simulink model "HVDCMTGW"  (R2025b)
settings: Solver=VariableStepAuto  StartTime=0.0  StopTime=Tsim  FixedStep=5e-5  RelTol=1e-3
PreLoadFcn:
  | SimulationTime = 3.5;
  | HVDCParameters;
  | Tsim = 3.5;
undefined symbols (not defined in the file): base, Base, Connection1, Connection2, Connection3, DiscIntNeverNeededParam, ee_sli_rtmsupport, frt, gcbh, grid, HVDC, lvrt, onshoreGfm, pll, pmsm, PVController, time, Ts, windController, windTransformer, windTurbine
libraries: fl_lib x51, ee_lib x46, nesl_utility x41, simulink x18, eeGeneralControl x12, eeTransforms x6
(part 3 of 4)

== system HVDCMTGW/HVDC STATION 3/GFM Control/Subsystem3 ==
  Current Sensor : fl_lib/Electrical/Electrical Sensors/Current Sensor
  Voltage Sensor1 : fl_lib/Electrical/Electrical Sensors/Voltage Sensor
  - : PMIOPort  Side=Left
  Idc : PMIOPort  Port=2  Side=Right
  Vdc : PMIOPort  Port=3  Side=Right
  + : PMIOPort  Port=4  Side=Right
  Ref : PMIOPort  Port=5  Side=Right
  connections:
  Current Sensor/LConn1 -- Voltage Sensor1/LConn1 -- +/RConn1
  Idc/RConn1 -- Current Sensor/RConn1
  Voltage Sensor1/RConn1 -- Vdc/RConn1
  Voltage Sensor1/RConn2 -- Ref/RConn1
  Current Sensor/RConn2 -- -/RConn1

== system HVDCMTGW/Wind Farm 1/PLL & Measurements/Measurement1 ==
  u : Inport
  Ig : Outport
  wires:
  u/1 -> Ig/1

== system HVDCMTGW/Wind Farm 1/PLL & Measurements/Measurement2 ==
  u : Inport
  Vg : Outport
  wires:
  u/1 -> Vg/1

== system HVDCMTGW/Wind Farm 1/PLL & Measurements/PLL ==
  abc : Inport
  Ig : Inport  Port=2
  Demux : Demux  Outputs=3
  Demux1 : Demux  Outputs=3
  Park Transform : eeTransforms/Park Transform  AxisAlignment=Q-axis  PowerInvariant=off
  Park Transform1 : eeTransforms/Park Transform  AxisAlignment=Q-axis  PowerInvariant=off
  "Sinusoidal Measurement (PLL, Three-Phase)1" : Subsystem  LoadFcn=ee_sli_rtmsupport( 'loadfcn', gcbh );  mask(Sinusoidal Measurement (PLL, Three-Phase)){Kp_LF=pll.kp, Ki_LF=pll.ki*0.25, F0=grid.frequency, Theta0=0, Ts=Ts}
      mask prompts: Kp_LF "physmod:ee:library:comments:control:eeSinusoidalMeasurement:LoopFilterProportionalGain_MP"; Ki_LF "physmod:ee:library:comments:control:eeSinusoidalMeasurement:LoopFilterIntegralGain_MP"; F0 "physmod:ee:library:comments:control:eeSinusoidalMeasurement:InitialFrequencyHz_MP"; Theta0 "physmod:ee:library:comments:control:eeSinusoidalMeasurement:InitialPhaseAnglerad_MP"; Ts "physmod:ee:library:comments:control:eeSinusoidalMeasurement:SampleTime1ForInherited_MP"
      mask help: physmod:ee:library:comments:control:eeSinusoidalMeasurement:SinusoidalPowerMeasurementPLLThreePhase_MD
      mask init:
      | timeDomain = ee.mask.initializeThreePhaseSinusoidalMeasurementPLL(Ts);
      settings: CopyFcn=ee_sli_rtmsupport( 'copyfcn', gcbh );  DeleteFcn=ee_sli_rtmsupport( 'deletefcn', gcbh );  ModelCloseFcn=ee_sli_rtmsupport( 'modelclosefcn', gcbh );  PostSaveFcn=ee_sli_rtmsupport( 'postsavefcn', gcbh );  PreCopyFcn=ee_sli_rtmsupport( 'precopyfcn', gcbh );  OpenFcn=ee_sli_rtmsupport( 'openfcn', gcbh );  CloseFcn=ee_sli_rtmsupport( 'closefcn', gcbh );  PreDeleteFcn=ee_sli_rtmsupport( 'predeletefcn', gcbh );
      settings: LibrarySourceBlock=|
      | ee_sl_lib/Measurements/Sinusoidal Measurement
      | (PLL, Three-Phase)
      mask Help: web(nesl_help(gcbh))
      mask TypeOptions Ts:
      | Angle/Integrator with
      | Wrapped State
      | (Discrete or Continuous)/Ts | PI/Integrator
      | (Discrete or Continuous)/Ts | Moving Average
      | (Variable Frequency)/Ts | Low-Pass Filter
      | (Discrete or Continuous)/Ts
      mask DialogControl Kp_LF Prompt: Loop filter proportional gain
      mask DialogControl Ki_LF Prompt: Loop filter integral gain
      mask DialogControl F0 Prompt: Initial frequency (Hz)
      mask DialogControl Theta0 Prompt: Initial phase angle (rad)
      mask DialogControl Ts Prompt: Sample time (-1 for inherited)
      mask Display: ee.mask.drawThreePhaseSinusoidalMeasurementPLL;
  Terminator : Terminator
  Terminator1 : Terminator
  abc1 : InportShadow
  mag : Outport
  freq : Outport  Port=2
  angle : Outport  Port=3
  Vd : Outport  Port=4
  Vq : Outport  Port=5
  Id : Outport  Port=6
  Iq : Outport  Port=7
  wires:
  Demux/3 -> Terminator/1
  Park Transform/1 -> Demux/1
  Demux/1 -> Vd/1
  Demux/2 -> Vq/1
  "Sinusoidal Measurement (PLL, Three-Phase)1"/3(mag) -> mag/1
  "Sinusoidal Measurement (PLL, Three-Phase)1"/2(angle) -> angle/1, Park Transform/2, Park Transform1/2
  Ig/1 -> Park Transform1/1
  Demux1/2 -> Iq/1
  Park Transform1/1 -> Demux1/1
  Demux1/1 -> Id/1
  Demux1/3 -> Terminator1/1
  abc1/1 -> Park Transform/1
  abc/1 -> "Sinusoidal Measurement (PLL, Three-Phase)1"/1(abc)
  "Sinusoidal Measurement (PLL, Three-Phase)1"/1(freq) -> freq/1

== system HVDCMTGW/Wind Farm 1/Wind Farm/Abstract ==
  Vbus : Inport
  33/4.16 kV : ee_lib/Passive/Transformers/Two-Winding Transformer (Three-Phase)  SRated=windTransformer.va A*V  FRated=grid.frequency Hz  Winding1Connection=ee.enum.windingconnection.Yg  VRated1=windTransformer.hv1 V  Winding2Connection=ee.enum.windingconnection.Yg  VRated2=4.16e3 V  CoreType=ee.enum.coretype.threelimb  pu_Rw1=windTransformer.windingResistance/20  pu_Rw2=windTransformer.windingResistance/20  leakage_reactance_option=ee.enum.transformer_leakage.include  pu_Xl1=windTransformer.windingLekageReactance/20  pu_Xl2=windTransformer.windingLekageReactance/20  magnetizing_resistance_option=ee.enum.transformer_magnetizingResistance.exclude  pu_Rm=500  magnetizing_reactance_option=ee.enum.transformer_magnetizingReactance.exclude  saturation_option=ee.enum.transformer_saturation.exclude  pu_Xm=500  current_data=[0, .002, 1, 2]  magnetic_flux_data=[0, 1.2, 1.5, 1.51]  pu_X0=windTransformer.zeroSequenceReactance  i1_specify=off  i1_priority=None  i1=[0, 0, 0] A  i1_nominal_specify=off  i1_nominal_value=1  i1_nominal_unit=A  i2_specify=off  i2_priority=None  i2=[0, 0, 0] A  i2_nominal_specify=off  i2_nominal_value=1  i2_nominal_unit=A  phi_specify=off  phi_priority=None  phi=[0, 0, 0]  phi_nominal_specify=off  phi_nominal_value=1  phi_nominal_unit=1  power_dissipated_specify=off  power_dissipated_priority=None  power_dissipated=0 W  power_dissipated_nominal_specify=off  power_dissipated_nominal_value=1  power_dissipated_nominal_unit=W
      settings: InternalSimscapePortConfiguration="{\"Bottom\":[],\"Left\":[{\"id\":\"N1\",\"label\":\"~1\",\"type\":\"foundation.electrical.three_phase\"}],\"Right\":[{\"id\":\"N2\",\"label\":\"~2\",\"type\":\"foundation.electrical.three_phase\"}],\"Top\":[]}"
  Controlled Current Source (Three-Phase) : ee_lib/Sources/Controlled Current Source (Three-Phase)  input_option=ee.enum.inputType.instantaneous  FRated=60 Hz
      settings: InternalSimscapePortConfiguration="{\"Bottom\":[],\"Left\":[{\"id\":\"S\",\"label\":\"S\",\"type\":\"input\"},{\"id\":\"n\",\"label\":\"n\",\"type\":\"foundation.electrical.electrical\"}],\"Right\":[{\"id\":\"N\",\"label\":\"~\",\"type\":\"foundation.electrical.three_phase\"}],\"Top\":[]}"
  Current Sensor (Three-Phase) : ee_lib/Sensors & Transducers/Current Sensor (Three-Phase)
  Electrical Reference : fl_lib/Electrical/Electrical Elements/Electrical Reference
  POI : ee_lib/Sensors & Transducers/Current and Voltage Sensor (Three-Phase)  vMeasurementType=ee.enum.vmeasurement.ll  outputUnit=ee.enum.unit.pu  SRated=base.mVA A*V  VRated=base.kV V  I_specify=off  I_priority=None  I=[0, 0, 0] A  I_nominal_specify=off  I_nominal_value=1  I_nominal_unit=A  V_specify=off  V_priority=None  V=[0, 0, 0] V  V_nominal_specify=off  V_nominal_value=1  V_nominal_unit=V
      settings: InternalSimscapePortConfiguration="{\"Bottom\":[],\"Left\":[{\"id\":\"N1\",\"label\":\"~1\",\"type\":\"foundation.electrical.three_phase\"}],\"Right\":[{\"id\":\"V_output\",\"label\":\"V\",\"type\":\"output\"},{\"id\":\"I_output\",\"label\":\"I\",\"type\":\"output\"},{\"id\":\"N2\",\"label\":\"~2\",\"type\":\"foundation.electrical.three_phase\"}],\"Top\":[]}"
  PS Gain : fl_lib/Physical Signals/Functions/PS Gain  gain=2
  PS-Simulink Converter1 : nesl_utility/PS-Simulink Converter  PhysicalDomain=network_engine_domain  SubClassName=ps_output  LeftPortType=input  RightPortType=output  PseudoPeriodic=off  Frequencies=[]  VectorFormat=inherit  Unit=inherit  AffineConversion=off
  PS-Simulink Converter4 : nesl_utility/PS-Simulink Converter  PhysicalDomain=network_engine_domain  SubClassName=ps_output  LeftPortType=input  RightPortType=output  PseudoPeriodic=off  Frequencies=[]  VectorFormat=inherit  Unit=inherit  AffineConversion=off
  Wind Farm2 : Subsystem
  abc : PMIOPort  Side=Right
  abc1 : PMIOPort  Port=2  Side=Right
  Vabc : Outport
  Iabc : Outport  Port=2
  wires:
  Vbus/1 -> Wind Farm2/1(Vbus)
  PS-Simulink Converter1/1 -> Vabc/1  "Vabc"
  PS-Simulink Converter4/1 -> Iabc/1  "Iabc"
  connections:
  PS Gain/RConn1 -- Controlled Current Source (Three-Phase)/LConn1
  abc/RConn1 -- Current Sensor (Three-Phase)/RConn2
  Electrical Reference/LConn1 -- Controlled Current Source (Three-Phase)/LConn2
  PS-Simulink Converter1/LConn1 -- POI/RConn1
  PS-Simulink Converter4/LConn1 -- POI/RConn2
  33/4.16 kV/RConn1 -- POI/RConn3
  Current Sensor (Three-Phase)/LConn1 -- 33/4.16 kV/LConn1
  PS Gain/LConn1 -- Current Sensor (Three-Phase)/RConn1
  Wind Farm2/RConn1 -- POI/LConn1
  abc1/RConn1 -- Controlled Current Source (Three-Phase)/RConn1

== system HVDCMTGW/Wind Farm 1/Wind Farm/Detail ==
  Vbus : Inport
  33/4.16 kV : ee_lib/Passive/Transformers/Two-Winding Transformer (Three-Phase)  SRated=windTransformer.va A*V  FRated=grid.frequency Hz  Winding1Connection=ee.enum.windingconnection.Yg  VRated1=windTransformer.hv1 V  Winding2Connection=ee.enum.windingconnection.Yg  VRated2=4.16e3 V  CoreType=ee.enum.coretype.threelimb  pu_Rw1=windTransformer.windingResistance/20  pu_Rw2=windTransformer.windingResistance/20  leakage_reactance_option=ee.enum.transformer_leakage.include  pu_Xl1=windTransformer.windingLekageReactance/20  pu_Xl2=windTransformer.windingLekageReactance/20  magnetizing_resistance_option=ee.enum.transformer_magnetizingResistance.exclude  pu_Rm=500  magnetizing_reactance_option=ee.enum.transformer_magnetizingReactance.exclude  saturation_option=ee.enum.transformer_saturation.exclude  pu_Xm=500  current_data=[0, .002, 1, 2]  magnetic_flux_data=[0, 1.2, 1.5, 1.51]  pu_X0=windTransformer.zeroSequenceReactance  i1_specify=off  i1_priority=None  i1=[0, 0, 0] A  i1_nominal_specify=off  i1_nominal_value=1  i1_nominal_unit=A  i2_specify=off  i2_priority=None  i2=[0, 0, 0] A  i2_nominal_specify=off  i2_nominal_value=1  i2_nominal_unit=A  phi_specify=off  phi_priority=None  phi=[0, 0, 0]  phi_nominal_specify=off  phi_nominal_value=1  phi_nominal_unit=1  power_dissipated_specify=off  power_dissipated_priority=None  power_dissipated=0 W  power_dissipated_nominal_specify=off  power_dissipated_nominal_value=1  power_dissipated_nominal_unit=W
      settings: InternalSimscapePortConfiguration="{\"Bottom\":[],\"Left\":[{\"id\":\"N1\",\"label\":\"~1\",\"type\":\"foundation.electrical.three_phase\"}],\"Right\":[{\"id\":\"N2\",\"label\":\"~2\",\"type\":\"foundation.electrical.three_phase\"}],\"Top\":[]}"
  33/4.16 kV1 : ee_lib/Passive/Transformers/Two-Winding Transformer (Three-Phase)  SRated=windTransformer.va A*V  FRated=grid.frequency Hz  Winding1Connection=ee.enum.windingconnection.Yg  VRated1=windTransformer.hv1 V  Winding2Connection=ee.enum.windingconnection.Yg  VRated2=4.16e3 V  CoreType=ee.enum.coretype.threelimb  pu_Rw1=windTransformer.windingResistance/20  pu_Rw2=windTransformer.windingResistance/20  leakage_reactance_option=ee.enum.transformer_leakage.include  pu_Xl1=windTransformer.windingLekageReactance/20  pu_Xl2=windTransformer.windingLekageReactance/20  magnetizing_resistance_option=ee.enum.transformer_magnetizingResistance.exclude  pu_Rm=500  magnetizing_reactance_option=ee.enum.transformer_magnetizingReactance.exclude  saturation_option=ee.enum.transformer_saturation.exclude  pu_Xm=500  current_data=[0, .002, 1, 2]  magnetic_flux_data=[0, 1.2, 1.5, 1.51]  pu_X0=windTransformer.zeroSequenceReactance  i1_specify=off  i1_priority=None  i1=[0, 0, 0] A  i1_nominal_specify=off  i1_nominal_value=1  i1_nominal_unit=A  i2_specify=off  i2_priority=None  i2=[0, 0, 0] A  i2_nominal_specify=off  i2_nominal_value=1  i2_nominal_unit=A  phi_specify=off  phi_priority=None  phi=[0, 0, 0]  phi_nominal_specify=off  phi_nominal_value=1  phi_nominal_unit=1  power_dissipated_specify=off  power_dissipated_priority=None  power_dissipated=0 W  power_dissipated_nominal_specify=off  power_dissipated_nominal_value=1  power_dissipated_nominal_unit=W
      settings: InternalSimscapePortConfiguration="{\"Bottom\":[],\"Left\":[{\"id\":\"N1\",\"label\":\"~1\",\"type\":\"foundation.electrical.three_phase\"}],\"Right\":[{\"id\":\"N2\",\"label\":\"~2\",\"type\":\"foundation.electrical.three_phase\"}],\"Top\":[]}"
  POI : ee_lib/Sensors & Transducers/Current and Voltage Sensor (Three-Phase)  vMeasurementType=ee.enum.vmeasurement.ll  outputUnit=ee.enum.unit.pu  SRated=base.mVA A*V  VRated=base.kV V  I_specify=off  I_priority=None  I=[0, 0, 0] A  I_nominal_specify=off  I_nominal_value=1  I_nominal_unit=A  V_specify=off  V_priority=None  V=[0, 0, 0] V  V_nominal_specify=off  V_nominal_value=1  V_nominal_unit=V
      settings: InternalSimscapePortConfiguration="{\"Bottom\":[],\"Left\":[{\"id\":\"N1\",\"label\":\"~1\",\"type\":\"foundation.electrical.three_phase\"}],\"Right\":[{\"id\":\"V_output\",\"label\":\"V\",\"type\":\"output\"},{\"id\":\"I_output\",\"label\":\"I\",\"type\":\"output\"},{\"id\":\"N2\",\"label\":\"~2\",\"type\":\"foundation.electrical.three_phase\"}],\"Top\":[]}"
  PS-Simulink Converter1 : nesl_utility/PS-Simulink Converter  PhysicalDomain=network_engine_domain  SubClassName=ps_output  LeftPortType=input  RightPortType=output  PseudoPeriodic=off  Frequencies=[]  VectorFormat=inherit  Unit=inherit  AffineConversion=off
  PS-Simulink Converter4 : nesl_utility/PS-Simulink Converter  PhysicalDomain=network_engine_domain  SubClassName=ps_output  LeftPortType=input  RightPortType=output  PseudoPeriodic=off  Frequencies=[]  VectorFormat=inherit  Unit=inherit  AffineConversion=off
  Wind Farm1 : Subsystem
  Wind Farm2 : Subsystem
  Wind Farm3 : Subsystem
  abc : PMIOPort  Side=Right
  abc1 : PMIOPort  Port=2  Side=Right
  Vabc : Outport
  Iabc : Outport  Port=2
  wires:
  Vbus/1 -> Wind Farm3/1(Vbus), Wind Farm2/1(Vbus), Wind Farm1/1(Vbus)
  PS-Simulink Converter4/1 -> Iabc/1  "Iabc"
  PS-Simulink Converter1/1 -> Vabc/1  "Vabc"
  connections:
  Wind Farm2/RConn1 -- Wind Farm1/RConn1 -- POI/LConn1 -- Wind Farm3/RConn1
  abc/RConn1 -- 33/4.16 kV/LConn1
  PS-Simulink Converter4/LConn1 -- POI/RConn2
  PS-Simulink Converter1/LConn1 -- POI/RConn1
  POI/RConn3 -- 33/4.16 kV1/RConn1 -- 33/4.16 kV/RConn1
  abc1/RConn1 -- 33/4.16 kV1/LConn1

== system HVDCMTGW/Wind Farm 2/PLL & Measurements/Measurement1 ==
  u : Inport
  Ig : Outport
  wires:
  u/1 -> Ig/1

== system HVDCMTGW/Wind Farm 2/PLL & Measurements/Measurement2 ==
  u : Inport
  Vg : Outport
  wires:
  u/1 -> Vg/1

== system HVDCMTGW/Wind Farm 2/PLL & Measurements/PLL ==
  abc : Inport
  Ig : Inport  Port=2
  Demux : Demux  Outputs=3
  Demux1 : Demux  Outputs=3
  Park Transform : eeTransforms/Park Transform  AxisAlignment=Q-axis  PowerInvariant=off
  Park Transform1 : eeTransforms/Park Transform  AxisAlignment=Q-axis  PowerInvariant=off
  "Sinusoidal Measurement (PLL, Three-Phase)1" : Subsystem  LoadFcn=ee_sli_rtmsupport( 'loadfcn', gcbh );  mask(Sinusoidal Measurement (PLL, Three-Phase)){Kp_LF=pll.kp, Ki_LF=pll.ki*0.25, F0=grid.frequency, Theta0=0, Ts=Ts}
      mask prompts: Kp_LF "physmod:ee:library:comments:control:eeSinusoidalMeasurement:LoopFilterProportionalGain_MP"; Ki_LF "physmod:ee:library:comments:control:eeSinusoidalMeasurement:LoopFilterIntegralGain_MP"; F0 "physmod:ee:library:comments:control:eeSinusoidalMeasurement:InitialFrequencyHz_MP"; Theta0 "physmod:ee:library:comments:control:eeSinusoidalMeasurement:InitialPhaseAnglerad_MP"; Ts "physmod:ee:library:comments:control:eeSinusoidalMeasurement:SampleTime1ForInherited_MP"
      mask help: physmod:ee:library:comments:control:eeSinusoidalMeasurement:SinusoidalPowerMeasurementPLLThreePhase_MD
      mask init:
      | timeDomain = ee.mask.initializeThreePhaseSinusoidalMeasurementPLL(Ts);
      settings: CopyFcn=ee_sli_rtmsupport( 'copyfcn', gcbh );  DeleteFcn=ee_sli_rtmsupport( 'deletefcn', gcbh );  ModelCloseFcn=ee_sli_rtmsupport( 'modelclosefcn', gcbh );  PostSaveFcn=ee_sli_rtmsupport( 'postsavefcn', gcbh );  PreCopyFcn=ee_sli_rtmsupport( 'precopyfcn', gcbh );  OpenFcn=ee_sli_rtmsupport( 'openfcn', gcbh );  CloseFcn=ee_sli_rtmsupport( 'closefcn', gcbh );  PreDeleteFcn=ee_sli_rtmsupport( 'predeletefcn', gcbh );
      settings: LibrarySourceBlock=|
      | ee_sl_lib/Measurements/Sinusoidal Measurement
      | (PLL, Three-Phase)
      mask Help: web(nesl_help(gcbh))
      mask TypeOptions Ts:
      | Angle/Integrator with
      | Wrapped State
      | (Discrete or Continuous)/Ts | PI/Integrator
      | (Discrete or Continuous)/Ts | Moving Average
      | (Variable Frequency)/Ts | Low-Pass Filter
      | (Discrete or Continuous)/Ts
      mask DialogControl Kp_LF Prompt: Loop filter proportional gain
      mask DialogControl Ki_LF Prompt: Loop filter integral gain
      mask DialogControl F0 Prompt: Initial frequency (Hz)
      mask DialogControl Theta0 Prompt: Initial phase angle (rad)
      mask DialogControl Ts Prompt: Sample time (-1 for inherited)
      mask Display: ee.mask.drawThreePhaseSinusoidalMeasurementPLL;
  Terminator : Terminator
  Terminator1 : Terminator
  abc1 : InportShadow
  mag : Outport
  freq : Outport  Port=2
  angle : Outport  Port=3
  Vd : Outport  Port=4
  Vq : Outport  Port=5
  Id : Outport  Port=6
  Iq : Outport  Port=7
  wires:
  Demux/3 -> Terminator/1
  Park Transform/1 -> Demux/1
  Demux/1 -> Vd/1
  Demux/2 -> Vq/1
  "Sinusoidal Measurement (PLL, Three-Phase)1"/3(mag) -> mag/1
  "Sinusoidal Measurement (PLL, Three-Phase)1"/2(angle) -> angle/1, Park Transform/2, Park Transform1/2
  Ig/1 -> Park Transform1/1
  Demux1/2 -> Iq/1
  Park Transform1/1 -> Demux1/1
  Demux1/1 -> Id/1
  Demux1/3 -> Terminator1/1
  abc1/1 -> Park Transform/1
  abc/1 -> "Sinusoidal Measurement (PLL, Three-Phase)1"/1(abc)
  "Sinusoidal Measurement (PLL, Three-Phase)1"/1(freq) -> freq/1

== system HVDCMTGW/Wind Farm 2/Wind Farm/Abstract ==
  Vbus : Inport
  33/4.16 kV : ee_lib/Passive/Transformers/Two-Winding Transformer (Three-Phase)  SRated=windTransformer.va A*V  FRated=grid.frequency Hz  Winding1Connection=ee.enum.windingconnection.Yg  VRated1=windTransformer.hv1 V  Winding2Connection=ee.enum.windingconnection.Yg  VRated2=4.16e3 V  CoreType=ee.enum.coretype.threelimb  pu_Rw1=windTransformer.windingResistance/20  pu_Rw2=windTransformer.windingResistance/20  leakage_reactance_option=ee.enum.transformer_leakage.include  pu_Xl1=windTransformer.windingLekageReactance/20  pu_Xl2=windTransformer.windingLekageReactance/20  magnetizing_resistance_option=ee.enum.transformer_magnetizingResistance.exclude  pu_Rm=500  magnetizing_reactance_option=ee.enum.transformer_magnetizingReactance.exclude  saturation_option=ee.enum.transformer_saturation.exclude  pu_Xm=500  current_data=[0, .002, 1, 2]  magnetic_flux_data=[0, 1.2, 1.5, 1.51]  pu_X0=windTransformer.zeroSequenceReactance  i1_specify=off  i1_priority=None  i1=[0, 0, 0] A  i1_nominal_specify=off  i1_nominal_value=1  i1_nominal_unit=A  i2_specify=off  i2_priority=None  i2=[0, 0, 0] A  i2_nominal_specify=off  i2_nominal_value=1  i2_nominal_unit=A  phi_specify=off  phi_priority=None  phi=[0, 0, 0]  phi_nominal_specify=off  phi_nominal_value=1  phi_nominal_unit=1  power_dissipated_specify=off  power_dissipated_priority=None  power_dissipated=0 W  power_dissipated_nominal_specify=off  power_dissipated_nominal_value=1  power_dissipated_nominal_unit=W
      settings: InternalSimscapePortConfiguration="{\"Bottom\":[],\"Left\":[{\"id\":\"N1\",\"label\":\"~1\",\"type\":\"foundation.electrical.three_phase\"}],\"Right\":[{\"id\":\"N2\",\"label\":\"~2\",\"type\":\"foundation.electrical.three_phase\"}],\"Top\":[]}"
  Controlled Current Source (Three-Phase) : ee_lib/Sources/Controlled Current Source (Three-Phase)  input_option=ee.enum.inputType.instantaneous  FRated=60 Hz
      settings: InternalSimscapePortConfiguration="{\"Bottom\":[],\"Left\":[{\"id\":\"S\",\"label\":\"S\",\"type\":\"input\"},{\"id\":\"n\",\"label\":\"n\",\"type\":\"foundation.electrical.electrical\"}],\"Right\":[{\"id\":\"N\",\"label\":\"~\",\"type\":\"foundation.electrical.three_phase\"}],\"Top\":[]}"
  Current Sensor (Three-Phase) : ee_lib/Sensors & Transducers/Current Sensor (Three-Phase)
  Electrical Reference : fl_lib/Electrical/Electrical Elements/Electrical Reference
  POI : ee_lib/Sensors & Transducers/Current and Voltage Sensor (Three-Phase)  vMeasurementType=ee.enum.vmeasurement.ll  outputUnit=ee.enum.unit.pu  SRated=base.mVA A*V  VRated=base.kV V  I_specify=off  I_priority=None  I=[0, 0, 0] A  I_nominal_specify=off  I_nominal_value=1  I_nominal_unit=A  V_specify=off  V_priority=None  V=[0, 0, 0] V  V_nominal_specify=off  V_nominal_value=1  V_nominal_unit=V
      settings: InternalSimscapePortConfiguration="{\"Bottom\":[],\"Left\":[{\"id\":\"N1\",\"label\":\"~1\",\"type\":\"foundation.electrical.three_phase\"}],\"Right\":[{\"id\":\"V_output\",\"label\":\"V\",\"type\":\"output\"},{\"id\":\"I_output\",\"label\":\"I\",\"type\":\"output\"},{\"id\":\"N2\",\"label\":\"~2\",\"type\":\"foundation.electrical.three_phase\"}],\"Top\":[]}"
  PS Gain : fl_lib/Physical Signals/Functions/PS Gain  gain=2
  PS-Simulink Converter1 : nesl_utility/PS-Simulink Converter  PhysicalDomain=network_engine_domain  SubClassName=ps_output  LeftPortType=input  RightPortType=output  PseudoPeriodic=off  Frequencies=[]  VectorFormat=inherit  Unit=inherit  AffineConversion=off
  PS-Simulink Converter4 : nesl_utility/PS-Simulink Converter  PhysicalDomain=network_engine_domain  SubClassName=ps_output  LeftPortType=input  RightPortType=output  PseudoPeriodic=off  Frequencies=[]  VectorFormat=inherit  Unit=inherit  AffineConversion=off
  Wind Farm2 : Subsystem
  abc : PMIOPort  Side=Right
  abc1 : PMIOPort  Port=2  Side=Right
  Vabc : Outport
  Iabc : Outport  Port=2
  wires:
  Vbus/1 -> Wind Farm2/1(Vbus)
  PS-Simulink Converter1/1 -> Vabc/1  "Vabc"
  PS-Simulink Converter4/1 -> Iabc/1  "Iabc"
  connections:
  PS Gain/RConn1 -- Controlled Current Source (Three-Phase)/LConn1
  abc/RConn1 -- Current Sensor (Three-Phase)/RConn2
  Electrical Reference/LConn1 -- Controlled Current Source (Three-Phase)/LConn2
  PS-Simulink Converter1/LConn1 -- POI/RConn1
  PS-Simulink Converter4/LConn1 -- POI/RConn2
  33/4.16 kV/RConn1 -- POI/RConn3
  Current Sensor (Three-Phase)/LConn1 -- 33/4.16 kV/LConn1
  PS Gain/LConn1 -- Current Sensor (Three-Phase)/RConn1
  Wind Farm2/RConn1 -- POI/LConn1
  abc1/RConn1 -- Controlled Current Source (Three-Phase)/RConn1

== system HVDCMTGW/Wind Farm 2/Wind Farm/Detail ==
  Vbus : Inport
  33/4.16 kV : ee_lib/Passive/Transformers/Two-Winding Transformer (Three-Phase)  SRated=windTransformer.va A*V  FRated=grid.frequency Hz  Winding1Connection=ee.enum.windingconnection.Yg  VRated1=windTransformer.hv1 V  Winding2Connection=ee.enum.windingconnection.Yg  VRated2=4.16e3 V  CoreType=ee.enum.coretype.threelimb  pu_Rw1=windTransformer.windingResistance/20  pu_Rw2=windTransformer.windingResistance/20  leakage_reactance_option=ee.enum.transformer_leakage.include  pu_Xl1=windTransformer.windingLekageReactance/20  pu_Xl2=windTransformer.windingLekageReactance/20  magnetizing_resistance_option=ee.enum.transformer_magnetizingResistance.exclude  pu_Rm=500  magnetizing_reactance_option=ee.enum.transformer_magnetizingReactance.exclude  saturation_option=ee.enum.transformer_saturation.exclude  pu_Xm=500  current_data=[0, .002, 1, 2]  magnetic_flux_data=[0, 1.2, 1.5, 1.51]  pu_X0=windTransformer.zeroSequenceReactance  i1_specify=off  i1_priority=None  i1=[0, 0, 0] A  i1_nominal_specify=off  i1_nominal_value=1  i1_nominal_unit=A  i2_specify=off  i2_priority=None  i2=[0, 0, 0] A  i2_nominal_specify=off  i2_nominal_value=1  i2_nominal_unit=A  phi_specify=off  phi_priority=None  phi=[0, 0, 0]  phi_nominal_specify=off  phi_nominal_value=1  phi_nominal_unit=1  power_dissipated_specify=off  power_dissipated_priority=None  power_dissipated=0 W  power_dissipated_nominal_specify=off  power_dissipated_nominal_value=1  power_dissipated_nominal_unit=W
      settings: InternalSimscapePortConfiguration="{\"Bottom\":[],\"Left\":[{\"id\":\"N1\",\"label\":\"~1\",\"type\":\"foundation.electrical.three_phase\"}],\"Right\":[{\"id\":\"N2\",\"label\":\"~2\",\"type\":\"foundation.electrical.three_phase\"}],\"Top\":[]}"
  33/4.16 kV1 : ee_lib/Passive/Transformers/Two-Winding Transformer (Three-Phase)  SRated=windTransformer.va A*V  FRated=grid.frequency Hz  Winding1Connection=ee.enum.windingconnection.Yg  VRated1=windTransformer.hv1 V  Winding2Connection=ee.enum.windingconnection.Yg  VRated2=4.16e3 V  CoreType=ee.enum.coretype.threelimb  pu_Rw1=windTransformer.windingResistance/20  pu_Rw2=windTransformer.windingResistance/20  leakage_reactance_option=ee.enum.transformer_leakage.include  pu_Xl1=windTransformer.windingLekageReactance/20  pu_Xl2=windTransformer.windingLekageReactance/20  magnetizing_resistance_option=ee.enum.transformer_magnetizingResistance.exclude  pu_Rm=500  magnetizing_reactance_option=ee.enum.transformer_magnetizingReactance.exclude  saturation_option=ee.enum.transformer_saturation.exclude  pu_Xm=500  current_data=[0, .002, 1, 2]  magnetic_flux_data=[0, 1.2, 1.5, 1.51]  pu_X0=windTransformer.zeroSequenceReactance  i1_specify=off  i1_priority=None  i1=[0, 0, 0] A  i1_nominal_specify=off  i1_nominal_value=1  i1_nominal_unit=A  i2_specify=off  i2_priority=None  i2=[0, 0, 0] A  i2_nominal_specify=off  i2_nominal_value=1  i2_nominal_unit=A  phi_specify=off  phi_priority=None  phi=[0, 0, 0]  phi_nominal_specify=off  phi_nominal_value=1  phi_nominal_unit=1  power_dissipated_specify=off  power_dissipated_priority=None  power_dissipated=0 W  power_dissipated_nominal_specify=off  power_dissipated_nominal_value=1  power_dissipated_nominal_unit=W
      settings: InternalSimscapePortConfiguration="{\"Bottom\":[],\"Left\":[{\"id\":\"N1\",\"label\":\"~1\",\"type\":\"foundation.electrical.three_phase\"}],\"Right\":[{\"id\":\"N2\",\"label\":\"~2\",\"type\":\"foundation.electrical.three_phase\"}],\"Top\":[]}"
  POI : ee_lib/Sensors & Transducers/Current and Voltage Sensor (Three-Phase)  vMeasurementType=ee.enum.vmeasurement.ll  outputUnit=ee.enum.unit.pu  SRated=base.mVA A*V  VRated=base.kV V  I_specify=off  I_priority=None  I=[0, 0, 0] A  I_nominal_specify=off  I_nominal_value=1  I_nominal_unit=A  V_specify=off  V_priority=None  V=[0, 0, 0] V  V_nominal_specify=off  V_nominal_value=1  V_nominal_unit=V
      settings: InternalSimscapePortConfiguration="{\"Bottom\":[],\"Left\":[{\"id\":\"N1\",\"label\":\"~1\",\"type\":\"foundation.electrical.three_phase\"}],\"Right\":[{\"id\":\"V_output\",\"label\":\"V\",\"type\":\"output\"},{\"id\":\"I_output\",\"label\":\"I\",\"type\":\"output\"},{\"id\":\"N2\",\"label\":\"~2\",\"type\":\"foundation.electrical.three_phase\"}],\"Top\":[]}"
  PS-Simulink Converter1 : nesl_utility/PS-Simulink Converter  PhysicalDomain=network_engine_domain  SubClassName=ps_output  LeftPortType=input  RightPortType=output  PseudoPeriodic=off  Frequencies=[]  VectorFormat=inherit  Unit=inherit  AffineConversion=off
  PS-Simulink Converter4 : nesl_utility/PS-Simulink Converter  PhysicalDomain=network_engine_domain  SubClassName=ps_output  LeftPortType=input  RightPortType=output  PseudoPeriodic=off  Frequencies=[]  VectorFormat=inherit  Unit=inherit  AffineConversion=off
  Wind Farm1 : Subsystem
  Wind Farm2 : Subsystem
  Wind Farm3 : Subsystem
  abc : PMIOPort  Side=Right
  abc1 : PMIOPort  Port=2  Side=Right
  Vabc : Outport
  Iabc : Outport  Port=2
  wires:
  Vbus/1 -> Wind Farm3/1(Vbus), Wind Farm2/1(Vbus), Wind Farm1/1(Vbus)
  PS-Simulink Converter4/1 -> Iabc/1  "Iabc"
  PS-Simulink Converter1/1 -> Vabc/1  "Vabc"
  connections:
  Wind Farm3/RConn1 -- POI/LConn1 -- Wind Farm2/RConn1 -- Wind Farm1/RConn1
  abc/RConn1 -- 33/4.16 kV/LConn1
  PS-Simulink Converter4/LConn1 -- POI/RConn2
  PS-Simulink Converter1/LConn1 -- POI/RConn1
  POI/RConn3 -- 33/4.16 kV1/RConn1 -- 33/4.16 kV/RConn1
  abc1/RConn1 -- 33/4.16 kV1/LConn1

== system HVDCMTGW/Wind Farm 1/PLL & Measurements/PLL/Sinusoidal Measurement (PLL, Three-Phase)1 ==
  note: Loop Filter (LF)
  note: Voltage-controlled oscillator (VCO)
  abc : Inport  PortDimensions=3  SampleTime=Ts
  Angle : Subsystem
  Low-Pass Filter (Discrete or Continuous) : eeGeneralControl/Low-Pass Filter (Discrete or Continuous)  K=1/2/pi  T=1e-3  B=inf  A=-inf  init_option=Specify as parameter  x0=F0  Ts=Ts
      settings: LibrarySourceBlock=|
      | eeSinusoidalMeasurementV2/Sinusoidal Measurement
      | (PLL, Three-Phase)/Low-Pass Filter
      | (Discrete or Continuous)
  Moving Average (Variable Frequency) : eeGeneralControl/Moving Average (Variable Frequency)  VariantControl=Variant1  LabelModeActiveChoice=Discrete  f0=F0  fmin=5  x0=0  BufferSize=8192  Ts=Ts
      settings: LibrarySourceBlock=|
      | eeSinusoidalMeasurementV2/Sinusoidal Measurement
      | (PLL, Three-Phase)/Moving Average
      | (Variable Frequency)
  PI : Subsystem
  Park Transform : eeTransforms/Park Transform  AxisAlignment=Q-axis  PowerInvariant=off
  Pythagorian Sum : Fcn  Expr=sqrt(u(1)^2+u(2)^2)
  Selector2 : Selector  InputPortWidth=3  IndexOptions=Index vector (dialog)  Indices=[2]  OutputSizes=1
  freq : Outport  VectorParamsAs1DForOutWhenUnconnected=off
  angle : Outport  Port=2  VectorParamsAs1DForOutWhenUnconnected=off
  mag : Outport  Port=3  VectorParamsAs1DForOutWhenUnconnected=off
  wires:
  Moving Average (Variable Frequency)/1 -> Selector2/1, Pythagorian Sum/1
  Selector2/1 -> PI/1(u)
  Low-Pass Filter (Discrete or Continuous)/1 -> freq/1, Moving Average (Variable Frequency)/1
  Angle/1(theta) -> angle/1, Park Transform/2
  PI/1(y) -> Angle/1(omega), Low-Pass Filter (Discrete or Continuous)/1
  Park Transform/1 -> Moving Average (Variable Frequency)/2
  Pythagorian Sum/1 -> mag/1
  abc/1 -> Park Transform/1

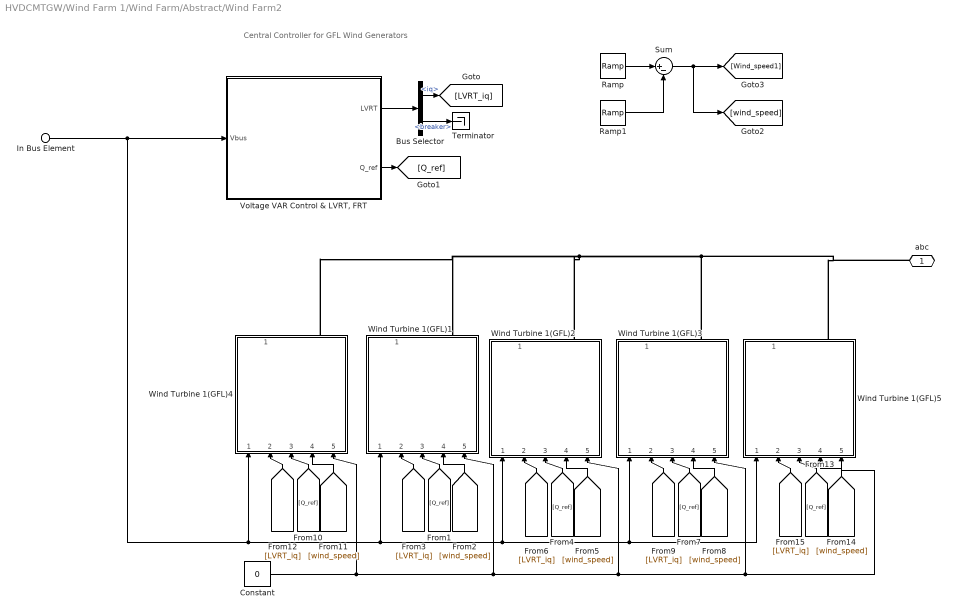
== system HVDCMTGW/Wind Farm 1/Wind Farm/Abstract/Wind Farm2 ==
  note: Central Controller for GFL Wind Generators
  In Bus Element : Inport  PortName=Vbus
  Bus Selector : BusSelector  OutputSignals=iq,breaker
  Constant : Constant  Value=0
  Ramp : simulink/Sources/Ramp  slope=-3  start=time.renewablevariation  InitialOutput=11
  Ramp1 : simulink/Sources/Ramp  slope=-3  start=time.renewablevariation+0.2  InitialOutput=0
  Sum : Sum  Inputs=|+-
  Terminator : Terminator
  "Voltage VAR Control & LVRT, FRT" : Subsystem
      mask Display: image('$imagefile'); % Use "Edit Image" on toolstrip to change.
  Wind Turbine 1(GFL){1..5} (5 alike) : Subsystem  ReferencedSubsystem=WindGFLMpp  p=pmsm.p  psim=pmsm.psim  Rs=pmsm.rs  Ld=pmsm.ld  Lq=pmsm.lq  Kdip_sm=pmsm.ld*pmsm.alpha  Kdii_sm=pmsm.rs*pmsm.alpha  Kqip_sm=pmsm.lq*pmsm.alpha  Kqii_sm=pmsm.rs*pmsm.alpha  airDensity=windTurbine.airDensity  turbineRadius=windTurbine.turbineRadius  pitch=windTurbine.pitch  TSR=windTurbine.TSR  cp=windTurbine.cp  wt=0.01  rt=0.01  Inertia=windTurbine.inertia  Kp_dc=windController.kpv  Ki_dc=windController.kiv  Kdpi_g=windController.kpic  Kdii_g=windController.kiic  Kqpi_g=windController.kpic  Kqii_g=windController.kiic  blk=Disabled  slop=2  tst=0
  abc : PMIOPort  Side=Right
  wires:
  Bus Selector/2 -> Terminator/1  "<breaker>"
  "Voltage VAR Control & LVRT, FRT"/1(LVRT) -> Bus Selector/1
  Ramp1/1 -> Sum/2
  Ramp/1 -> Sum/1
  [LVRT_iq] -> Wind Turbine 1(GFL)1/2
  [wind_speed] -> Wind Turbine 1(GFL)1/4
  [Q_ref] -> Wind Turbine 1(GFL)1/3
  Sum/1 -> [Wind_speed1], [wind_speed]
  [LVRT_iq] -> Wind Turbine 1(GFL)2/2
  [Q_ref] -> Wind Turbine 1(GFL)2/3
  [wind_speed] -> Wind Turbine 1(GFL)2/4
  [Q_ref] -> Wind Turbine 1(GFL)3/3
  [wind_speed] -> Wind Turbine 1(GFL)3/4
  [LVRT_iq] -> Wind Turbine 1(GFL)3/2
  In Bus Element/1 -> Wind Turbine 1(GFL)5/1, Wind Turbine 1(GFL)3/1, Wind Turbine 1(GFL)2/1, Wind Turbine 1(GFL)1/1, Wind Turbine 1(GFL)4/1, "Voltage VAR Control & LVRT, FRT"/1(Vbus)
  [LVRT_iq] -> Wind Turbine 1(GFL)4/2
  [Q_ref] -> Wind Turbine 1(GFL)4/3
  [wind_speed] -> Wind Turbine 1(GFL)4/4
  [LVRT_iq] -> Wind Turbine 1(GFL)5/2
  [Q_ref] -> Wind Turbine 1(GFL)5/3
  [wind_speed] -> Wind Turbine 1(GFL)5/4
  Bus Selector/1 -> [LVRT_iq]  "<iq>"
  "Voltage VAR Control & LVRT, FRT"/2(Q_ref) -> [Q_ref]
  Constant/1 -> Wind Turbine 1(GFL)5/5, Wind Turbine 1(GFL)3/5, Wind Turbine 1(GFL)2/5, Wind Turbine 1(GFL)1/5, Wind Turbine 1(GFL)4/5
  connections:
  Wind Turbine 1(GFL)3/RConn1 -- abc/RConn1 -- Wind Turbine 1(GFL)5/RConn1 -- Wind Turbine 1(GFL)2/RConn1 -- Wind Turbine 1(GFL)4/RConn1 -- Wind Turbine 1(GFL)1/RConn1

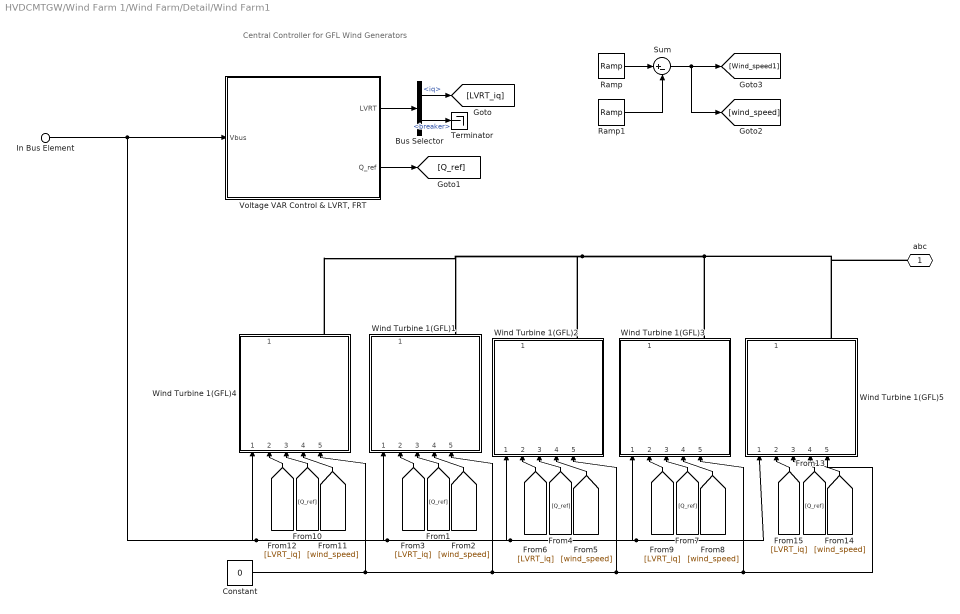
== system HVDCMTGW/Wind Farm 1/Wind Farm/Detail/Wind Farm1 ==
  note: Central Controller for GFL Wind Generators
  In Bus Element : Inport  PortName=Vbus
  Bus Selector : BusSelector  OutputSignals=iq,breaker
  Constant : Constant  Value=0
  Ramp : simulink/Sources/Ramp  slope=-3  start=time.renewablevariation  InitialOutput=11
  Ramp1 : simulink/Sources/Ramp  slope=-3  start=time.renewablevariation+0.2  InitialOutput=0
  Sum : Sum  Inputs=|+-
  Terminator : Terminator
  "Voltage VAR Control & LVRT, FRT" : Subsystem
      mask Display: image('$imagefile'); % Use "Edit Image" on toolstrip to change.
  Wind Turbine 1(GFL){1..5} (5 alike) : Subsystem  ReferencedSubsystem=WindGFLMpp  p=pmsm.p  psim=pmsm.psim  Rs=pmsm.rs  Ld=pmsm.ld  Lq=pmsm.lq  Kdip_sm=pmsm.ld*pmsm.alpha  Kdii_sm=pmsm.rs*pmsm.alpha  Kqip_sm=pmsm.lq*pmsm.alpha  Kqii_sm=pmsm.rs*pmsm.alpha  airDensity=windTurbine.airDensity  turbineRadius=windTurbine.turbineRadius  pitch=windTurbine.pitch  TSR=windTurbine.TSR  cp=windTurbine.cp  wt=0.01  rt=0.01  Inertia=windTurbine.inertia  Kp_dc=windController.kpv  Ki_dc=windController.kiv  Kdpi_g=windController.kpic  Kdii_g=windController.kiic  Kqpi_g=windController.kpic  Kqii_g=windController.kiic  blk=Enabled  slop=2  tst=0
  abc : PMIOPort  Side=Right
  wires:
  Bus Selector/2 -> Terminator/1  "<breaker>"
  "Voltage VAR Control & LVRT, FRT"/1(LVRT) -> Bus Selector/1
  Ramp1/1 -> Sum/2
  Ramp/1 -> Sum/1
  [LVRT_iq] -> Wind Turbine 1(GFL)1/2
  [wind_speed] -> Wind Turbine 1(GFL)1/4
  [Q_ref] -> Wind Turbine 1(GFL)1/3
  Sum/1 -> [Wind_speed1], [wind_speed]
  Bus Selector/1 -> [LVRT_iq]  "<iq>"
  "Voltage VAR Control & LVRT, FRT"/2(Q_ref) -> [Q_ref]
  [LVRT_iq] -> Wind Turbine 1(GFL)2/2
  [Q_ref] -> Wind Turbine 1(GFL)2/3
  [wind_speed] -> Wind Turbine 1(GFL)2/4
  [Q_ref] -> Wind Turbine 1(GFL)3/3
  [wind_speed] -> Wind Turbine 1(GFL)3/4
  [LVRT_iq] -> Wind Turbine 1(GFL)3/2
  In Bus Element/1 -> Wind Turbine 1(GFL)5/1, Wind Turbine 1(GFL)3/1, Wind Turbine 1(GFL)2/1, Wind Turbine 1(GFL)1/1, Wind Turbine 1(GFL)4/1, "Voltage VAR Control & LVRT, FRT"/1(Vbus)
  [LVRT_iq] -> Wind Turbine 1(GFL)4/2
  [Q_ref] -> Wind Turbine 1(GFL)4/3
  [wind_speed] -> Wind Turbine 1(GFL)4/4
  [LVRT_iq] -> Wind Turbine 1(GFL)5/2
  [Q_ref] -> Wind Turbine 1(GFL)5/3
  [wind_speed] -> Wind Turbine 1(GFL)5/4
  Constant/1 -> Wind Turbine 1(GFL)5/5, Wind Turbine 1(GFL)3/5, Wind Turbine 1(GFL)2/5, Wind Turbine 1(GFL)1/5, Wind Turbine 1(GFL)4/5
  connections:
  Wind Turbine 1(GFL)3/RConn1 -- abc/RConn1 -- Wind Turbine 1(GFL)5/RConn1 -- Wind Turbine 1(GFL)2/RConn1 -- Wind Turbine 1(GFL)4/RConn1 -- Wind Turbine 1(GFL)1/RConn1

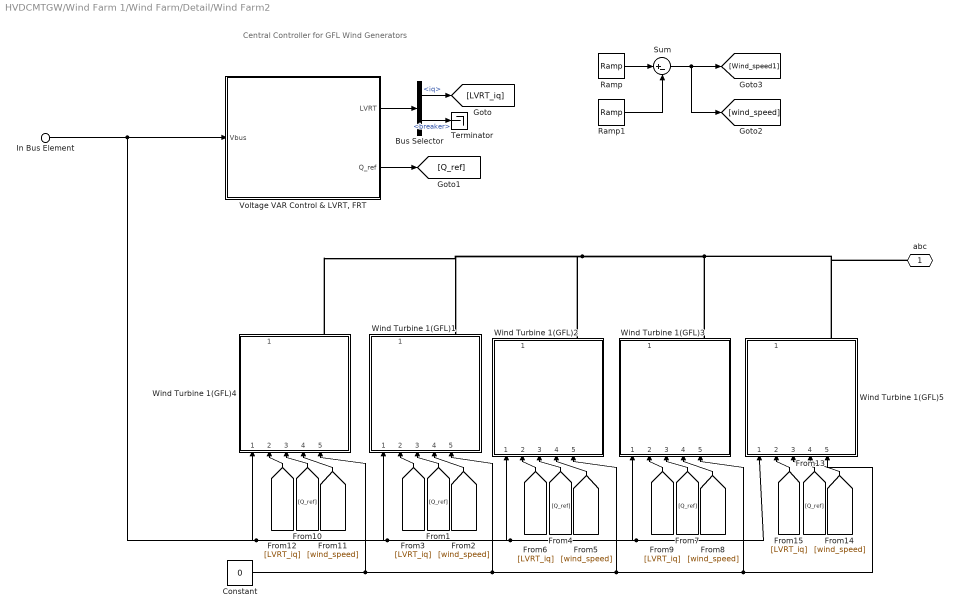
== system HVDCMTGW/Wind Farm 1/Wind Farm/Detail/Wind Farm2 ==
  note: Central Controller for GFL Wind Generators
  In Bus Element : Inport  PortName=Vbus
  Bus Selector : BusSelector  OutputSignals=iq,breaker
  Constant : Constant  Value=0
  Ramp : simulink/Sources/Ramp  slope=-3  start=time.renewablevariation  InitialOutput=11
  Ramp1 : simulink/Sources/Ramp  slope=-3  start=time.renewablevariation+0.2  InitialOutput=0
  Sum : Sum  Inputs=|+-
  Terminator : Terminator
  "Voltage VAR Control & LVRT, FRT" : Subsystem
      mask Display: image('$imagefile'); % Use "Edit Image" on toolstrip to change.
  Wind Turbine 1(GFL){1..5} (5 alike) : Subsystem  ReferencedSubsystem=WindGFLMpp  p=pmsm.p  psim=pmsm.psim  Rs=pmsm.rs  Ld=pmsm.ld  Lq=pmsm.lq  Kdip_sm=pmsm.ld*pmsm.alpha  Kdii_sm=pmsm.rs*pmsm.alpha  Kqip_sm=pmsm.lq*pmsm.alpha  Kqii_sm=pmsm.rs*pmsm.alpha  airDensity=windTurbine.airDensity  turbineRadius=windTurbine.turbineRadius  pitch=windTurbine.pitch  TSR=windTurbine.TSR  cp=windTurbine.cp  wt=0.01  rt=0.01  Inertia=windTurbine.inertia  Kp_dc=windController.kpv  Ki_dc=windController.kiv  Kdpi_g=windController.kpic  Kdii_g=windController.kiic  Kqpi_g=windController.kpic  Kqii_g=windController.kiic  blk=Enabled  slop=2  tst=0
  abc : PMIOPort  Side=Right
  wires:
  Bus Selector/2 -> Terminator/1  "<breaker>"
  "Voltage VAR Control & LVRT, FRT"/1(LVRT) -> Bus Selector/1
  Ramp1/1 -> Sum/2
  Ramp/1 -> Sum/1
  [LVRT_iq] -> Wind Turbine 1(GFL)1/2
  [wind_speed] -> Wind Turbine 1(GFL)1/4
  [Q_ref] -> Wind Turbine 1(GFL)1/3
  Sum/1 -> [Wind_speed1], [wind_speed]
  Bus Selector/1 -> [LVRT_iq]  "<iq>"
  "Voltage VAR Control & LVRT, FRT"/2(Q_ref) -> [Q_ref]
  [LVRT_iq] -> Wind Turbine 1(GFL)2/2
  [Q_ref] -> Wind Turbine 1(GFL)2/3
  [wind_speed] -> Wind Turbine 1(GFL)2/4
  [Q_ref] -> Wind Turbine 1(GFL)3/3
  [wind_speed] -> Wind Turbine 1(GFL)3/4
  [LVRT_iq] -> Wind Turbine 1(GFL)3/2
  In Bus Element/1 -> Wind Turbine 1(GFL)5/1, Wind Turbine 1(GFL)3/1, Wind Turbine 1(GFL)2/1, Wind Turbine 1(GFL)1/1, Wind Turbine 1(GFL)4/1, "Voltage VAR Control & LVRT, FRT"/1(Vbus)
  [LVRT_iq] -> Wind Turbine 1(GFL)4/2
  [Q_ref] -> Wind Turbine 1(GFL)4/3
  [wind_speed] -> Wind Turbine 1(GFL)4/4
  [LVRT_iq] -> Wind Turbine 1(GFL)5/2
  [Q_ref] -> Wind Turbine 1(GFL)5/3
  [wind_speed] -> Wind Turbine 1(GFL)5/4
  Constant/1 -> Wind Turbine 1(GFL)5/5, Wind Turbine 1(GFL)3/5, Wind Turbine 1(GFL)2/5, Wind Turbine 1(GFL)1/5, Wind Turbine 1(GFL)4/5
  connections:
  Wind Turbine 1(GFL)3/RConn1 -- abc/RConn1 -- Wind Turbine 1(GFL)5/RConn1 -- Wind Turbine 1(GFL)2/RConn1 -- Wind Turbine 1(GFL)4/RConn1 -- Wind Turbine 1(GFL)1/RConn1

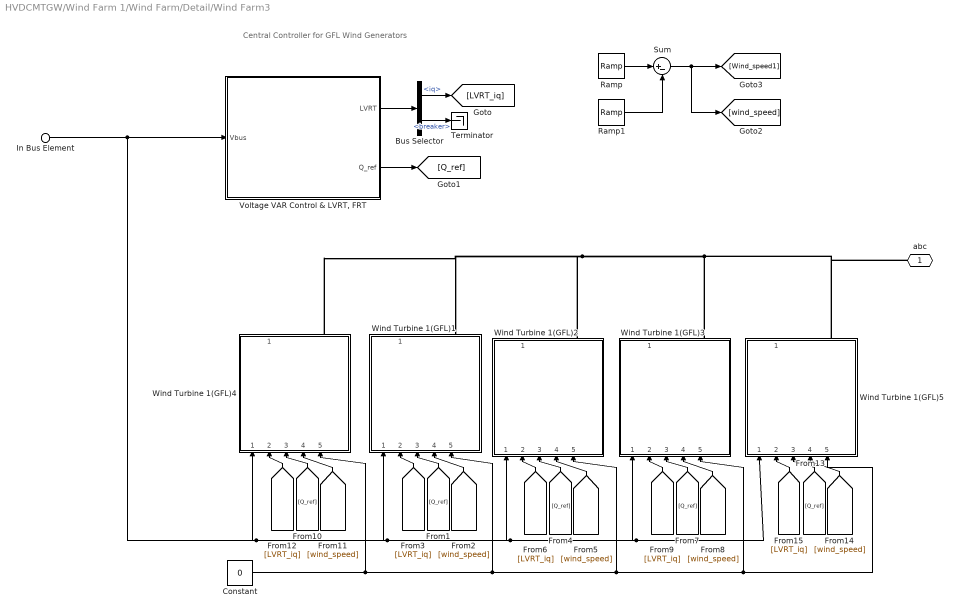
== system HVDCMTGW/Wind Farm 1/Wind Farm/Detail/Wind Farm3 ==
  note: Central Controller for GFL Wind Generators
  In Bus Element : Inport  PortName=Vbus
  Bus Selector : BusSelector  OutputSignals=iq,breaker
  Constant : Constant  Value=0
  Ramp : simulink/Sources/Ramp  slope=-3  start=time.renewablevariation  InitialOutput=11
  Ramp1 : simulink/Sources/Ramp  slope=-3  start=time.renewablevariation+0.2  InitialOutput=0
  Sum : Sum  Inputs=|+-
  Terminator : Terminator
  "Voltage VAR Control & LVRT, FRT" : Subsystem
      mask Display: image('$imagefile'); % Use "Edit Image" on toolstrip to change.
  Wind Turbine 1(GFL){1..5} (5 alike) : Subsystem  ReferencedSubsystem=WindGFLMpp  p=pmsm.p  psim=pmsm.psim  Rs=pmsm.rs  Ld=pmsm.ld  Lq=pmsm.lq  Kdip_sm=pmsm.ld*pmsm.alpha  Kdii_sm=pmsm.rs*pmsm.alpha  Kqip_sm=pmsm.lq*pmsm.alpha  Kqii_sm=pmsm.rs*pmsm.alpha  airDensity=windTurbine.airDensity  turbineRadius=windTurbine.turbineRadius  pitch=windTurbine.pitch  TSR=windTurbine.TSR  cp=windTurbine.cp  wt=0.01  rt=0.01  Inertia=windTurbine.inertia  Kp_dc=windController.kpv  Ki_dc=windController.kiv  Kdpi_g=windController.kpic  Kdii_g=windController.kiic  Kqpi_g=windController.kpic  Kqii_g=windController.kiic  blk=Enabled  slop=2  tst=0
  abc : PMIOPort  Side=Right
  wires:
  Bus Selector/2 -> Terminator/1  "<breaker>"
  "Voltage VAR Control & LVRT, FRT"/1(LVRT) -> Bus Selector/1
  Ramp1/1 -> Sum/2
  Ramp/1 -> Sum/1
  [LVRT_iq] -> Wind Turbine 1(GFL)1/2
  [wind_speed] -> Wind Turbine 1(GFL)1/4
  [Q_ref] -> Wind Turbine 1(GFL)1/3
  Sum/1 -> [Wind_speed1], [wind_speed]
  Bus Selector/1 -> [LVRT_iq]  "<iq>"
  "Voltage VAR Control & LVRT, FRT"/2(Q_ref) -> [Q_ref]
  [LVRT_iq] -> Wind Turbine 1(GFL)2/2
  [Q_ref] -> Wind Turbine 1(GFL)2/3
  [wind_speed] -> Wind Turbine 1(GFL)2/4
  [Q_ref] -> Wind Turbine 1(GFL)3/3
  [wind_speed] -> Wind Turbine 1(GFL)3/4
  [LVRT_iq] -> Wind Turbine 1(GFL)3/2
  In Bus Element/1 -> Wind Turbine 1(GFL)5/1, Wind Turbine 1(GFL)3/1, Wind Turbine 1(GFL)2/1, Wind Turbine 1(GFL)1/1, Wind Turbine 1(GFL)4/1, "Voltage VAR Control & LVRT, FRT"/1(Vbus)
  [LVRT_iq] -> Wind Turbine 1(GFL)4/2
  [Q_ref] -> Wind Turbine 1(GFL)4/3
  [wind_speed] -> Wind Turbine 1(GFL)4/4
  [LVRT_iq] -> Wind Turbine 1(GFL)5/2
  [Q_ref] -> Wind Turbine 1(GFL)5/3
  [wind_speed] -> Wind Turbine 1(GFL)5/4
  Constant/1 -> Wind Turbine 1(GFL)5/5, Wind Turbine 1(GFL)3/5, Wind Turbine 1(GFL)2/5, Wind Turbine 1(GFL)1/5, Wind Turbine 1(GFL)4/5
  connections:
  Wind Turbine 1(GFL)3/RConn1 -- abc/RConn1 -- Wind Turbine 1(GFL)5/RConn1 -- Wind Turbine 1(GFL)2/RConn1 -- Wind Turbine 1(GFL)4/RConn1 -- Wind Turbine 1(GFL)1/RConn1

== system HVDCMTGW/Wind Farm 2/PLL & Measurements/PLL/Sinusoidal Measurement (PLL, Three-Phase)1 ==
  note: Loop Filter (LF)
  note: Voltage-controlled oscillator (VCO)
  abc : Inport  PortDimensions=3  SampleTime=Ts
  Angle : Subsystem
  Low-Pass Filter (Discrete or Continuous) : eeGeneralControl/Low-Pass Filter (Discrete or Continuous)  K=1/2/pi  T=1e-3  B=inf  A=-inf  init_option=Specify as parameter  x0=F0  Ts=Ts
      settings: LibrarySourceBlock=|
      | eeSinusoidalMeasurementV2/Sinusoidal Measurement
      | (PLL, Three-Phase)/Low-Pass Filter
      | (Discrete or Continuous)
  Moving Average (Variable Frequency) : eeGeneralControl/Moving Average (Variable Frequency)  VariantControl=Variant1  LabelModeActiveChoice=Discrete  f0=F0  fmin=5  x0=0  BufferSize=8192  Ts=Ts
      settings: LibrarySourceBlock=|
      | eeSinusoidalMeasurementV2/Sinusoidal Measurement
      | (PLL, Three-Phase)/Moving Average
      | (Variable Frequency)
  PI : Subsystem
  Park Transform : eeTransforms/Park Transform  AxisAlignment=Q-axis  PowerInvariant=off
  Pythagorian Sum : Fcn  Expr=sqrt(u(1)^2+u(2)^2)
  Selector2 : Selector  InputPortWidth=3  IndexOptions=Index vector (dialog)  Indices=[2]  OutputSizes=1
  freq : Outport  VectorParamsAs1DForOutWhenUnconnected=off
  angle : Outport  Port=2  VectorParamsAs1DForOutWhenUnconnected=off
  mag : Outport  Port=3  VectorParamsAs1DForOutWhenUnconnected=off
  wires:
  Moving Average (Variable Frequency)/1 -> Selector2/1, Pythagorian Sum/1
  Selector2/1 -> PI/1(u)
  Low-Pass Filter (Discrete or Continuous)/1 -> freq/1, Moving Average (Variable Frequency)/1
  Angle/1(theta) -> angle/1, Park Transform/2
  PI/1(y) -> Angle/1(omega), Low-Pass Filter (Discrete or Continuous)/1
  Park Transform/1 -> Moving Average (Variable Frequency)/2
  Pythagorian Sum/1 -> mag/1
  abc/1 -> Park Transform/1

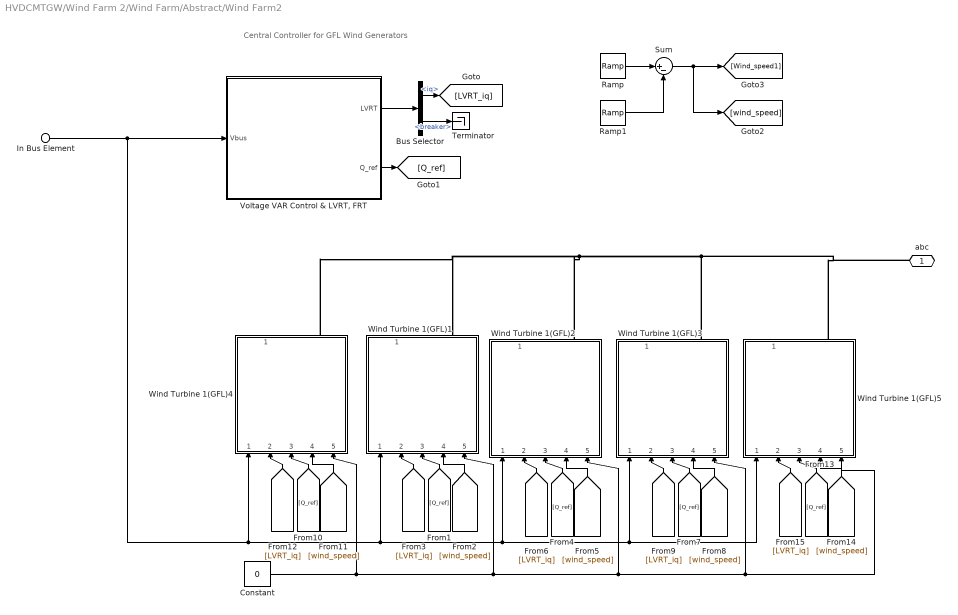
== system HVDCMTGW/Wind Farm 2/Wind Farm/Abstract/Wind Farm2 ==
  note: Central Controller for GFL Wind Generators
  In Bus Element : Inport  PortName=Vbus
  Bus Selector : BusSelector  OutputSignals=iq,breaker
  Constant : Constant  Value=0
  Ramp : simulink/Sources/Ramp  slope=-3  start=time.renewablevariation  InitialOutput=11
  Ramp1 : simulink/Sources/Ramp  slope=-3  start=time.renewablevariation+0.2  InitialOutput=0
  Sum : Sum  Inputs=|+-
  Terminator : Terminator
  "Voltage VAR Control & LVRT, FRT" : Subsystem
      mask Display: image('$imagefile'); % Use "Edit Image" on toolstrip to change.
  Wind Turbine 1(GFL){1..5} (5 alike) : Subsystem  ReferencedSubsystem=WindGFLMpp  p=pmsm.p  psim=pmsm.psim  Rs=pmsm.rs  Ld=pmsm.ld  Lq=pmsm.lq  Kdip_sm=pmsm.ld*pmsm.alpha  Kdii_sm=pmsm.rs*pmsm.alpha  Kqip_sm=pmsm.lq*pmsm.alpha  Kqii_sm=pmsm.rs*pmsm.alpha  airDensity=windTurbine.airDensity  turbineRadius=windTurbine.turbineRadius  pitch=windTurbine.pitch  TSR=windTurbine.TSR  cp=windTurbine.cp  wt=0.01  rt=0.01  Inertia=windTurbine.inertia  Kp_dc=windController.kpv  Ki_dc=windController.kiv  Kdpi_g=windController.kpic  Kdii_g=windController.kiic  Kqpi_g=windController.kpic  Kqii_g=windController.kiic  blk=Disabled  slop=2  tst=0
  abc : PMIOPort  Side=Right
  wires:
  Bus Selector/2 -> Terminator/1  "<breaker>"
  "Voltage VAR Control & LVRT, FRT"/1(LVRT) -> Bus Selector/1
  Ramp1/1 -> Sum/2
  Ramp/1 -> Sum/1
  [LVRT_iq] -> Wind Turbine 1(GFL)1/2
  [wind_speed] -> Wind Turbine 1(GFL)1/4
  [Q_ref] -> Wind Turbine 1(GFL)1/3
  Sum/1 -> [Wind_speed1], [wind_speed]
  [LVRT_iq] -> Wind Turbine 1(GFL)2/2
  [Q_ref] -> Wind Turbine 1(GFL)2/3
  [wind_speed] -> Wind Turbine 1(GFL)2/4
  [Q_ref] -> Wind Turbine 1(GFL)3/3
  [wind_speed] -> Wind Turbine 1(GFL)3/4
  [LVRT_iq] -> Wind Turbine 1(GFL)3/2
  In Bus Element/1 -> Wind Turbine 1(GFL)5/1, Wind Turbine 1(GFL)3/1, Wind Turbine 1(GFL)2/1, Wind Turbine 1(GFL)1/1, Wind Turbine 1(GFL)4/1, "Voltage VAR Control & LVRT, FRT"/1(Vbus)
  [LVRT_iq] -> Wind Turbine 1(GFL)4/2
  [Q_ref] -> Wind Turbine 1(GFL)4/3
  [wind_speed] -> Wind Turbine 1(GFL)4/4
  [LVRT_iq] -> Wind Turbine 1(GFL)5/2
  [Q_ref] -> Wind Turbine 1(GFL)5/3
  [wind_speed] -> Wind Turbine 1(GFL)5/4
  Bus Selector/1 -> [LVRT_iq]  "<iq>"
  "Voltage VAR Control & LVRT, FRT"/2(Q_ref) -> [Q_ref]
  Constant/1 -> Wind Turbine 1(GFL)5/5, Wind Turbine 1(GFL)3/5, Wind Turbine 1(GFL)2/5, Wind Turbine 1(GFL)1/5, Wind Turbine 1(GFL)4/5
  connections:
  Wind Turbine 1(GFL)3/RConn1 -- abc/RConn1 -- Wind Turbine 1(GFL)5/RConn1 -- Wind Turbine 1(GFL)2/RConn1 -- Wind Turbine 1(GFL)4/RConn1 -- Wind Turbine 1(GFL)1/RConn1

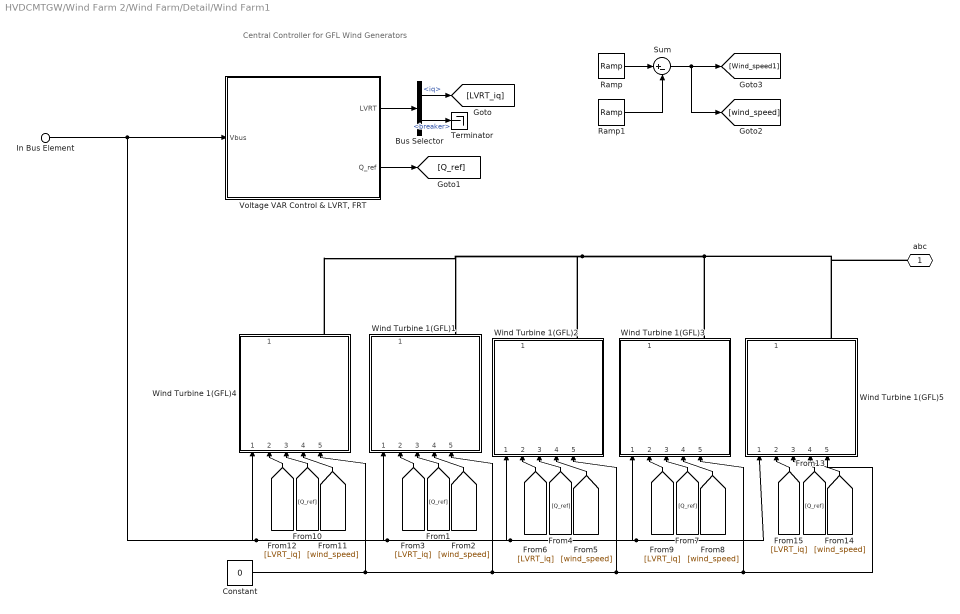
== system HVDCMTGW/Wind Farm 2/Wind Farm/Detail/Wind Farm1 ==
  note: Central Controller for GFL Wind Generators
  In Bus Element : Inport  PortName=Vbus
  Bus Selector : BusSelector  OutputSignals=iq,breaker
  Constant : Constant  Value=0
  Ramp : simulink/Sources/Ramp  slope=-3  start=time.renewablevariation  InitialOutput=11
  Ramp1 : simulink/Sources/Ramp  slope=-3  start=time.renewablevariation+0.2  InitialOutput=0
  Sum : Sum  Inputs=|+-
  Terminator : Terminator
  "Voltage VAR Control & LVRT, FRT" : Subsystem
      mask Display: image('$imagefile'); % Use "Edit Image" on toolstrip to change.
  Wind Turbine 1(GFL){1..5} (5 alike) : Subsystem  ReferencedSubsystem=WindGFLMpp  p=pmsm.p  psim=pmsm.psim  Rs=pmsm.rs  Ld=pmsm.ld  Lq=pmsm.lq  Kdip_sm=pmsm.ld*pmsm.alpha  Kdii_sm=pmsm.rs*pmsm.alpha  Kqip_sm=pmsm.lq*pmsm.alpha  Kqii_sm=pmsm.rs*pmsm.alpha  airDensity=windTurbine.airDensity  turbineRadius=windTurbine.turbineRadius  pitch=windTurbine.pitch  TSR=windTurbine.TSR  cp=windTurbine.cp  wt=0.01  rt=0.01  Inertia=windTurbine.inertia  Kp_dc=windController.kpv  Ki_dc=windController.kiv  Kdpi_g=windController.kpic  Kdii_g=windController.kiic  Kqpi_g=windController.kpic  Kqii_g=windController.kiic  blk=Enabled  slop=2  tst=0
  abc : PMIOPort  Side=Right
  wires:
  Bus Selector/2 -> Terminator/1  "<breaker>"
  "Voltage VAR Control & LVRT, FRT"/1(LVRT) -> Bus Selector/1
  Ramp1/1 -> Sum/2
  Ramp/1 -> Sum/1
  [LVRT_iq] -> Wind Turbine 1(GFL)1/2
  [wind_speed] -> Wind Turbine 1(GFL)1/4
  [Q_ref] -> Wind Turbine 1(GFL)1/3
  Sum/1 -> [Wind_speed1], [wind_speed]
  Bus Selector/1 -> [LVRT_iq]  "<iq>"
  "Voltage VAR Control & LVRT, FRT"/2(Q_ref) -> [Q_ref]
  [LVRT_iq] -> Wind Turbine 1(GFL)2/2
  [Q_ref] -> Wind Turbine 1(GFL)2/3
  [wind_speed] -> Wind Turbine 1(GFL)2/4
  [Q_ref] -> Wind Turbine 1(GFL)3/3
  [wind_speed] -> Wind Turbine 1(GFL)3/4
  [LVRT_iq] -> Wind Turbine 1(GFL)3/2
  In Bus Element/1 -> Wind Turbine 1(GFL)5/1, Wind Turbine 1(GFL)3/1, Wind Turbine 1(GFL)2/1, Wind Turbine 1(GFL)1/1, Wind Turbine 1(GFL)4/1, "Voltage VAR Control & LVRT, FRT"/1(Vbus)
  [LVRT_iq] -> Wind Turbine 1(GFL)4/2
  [Q_ref] -> Wind Turbine 1(GFL)4/3
  [wind_speed] -> Wind Turbine 1(GFL)4/4
  [LVRT_iq] -> Wind Turbine 1(GFL)5/2
  [Q_ref] -> Wind Turbine 1(GFL)5/3
  [wind_speed] -> Wind Turbine 1(GFL)5/4
  Constant/1 -> Wind Turbine 1(GFL)5/5, Wind Turbine 1(GFL)3/5, Wind Turbine 1(GFL)2/5, Wind Turbine 1(GFL)1/5, Wind Turbine 1(GFL)4/5
  connections:
  Wind Turbine 1(GFL)3/RConn1 -- abc/RConn1 -- Wind Turbine 1(GFL)5/RConn1 -- Wind Turbine 1(GFL)2/RConn1 -- Wind Turbine 1(GFL)4/RConn1 -- Wind Turbine 1(GFL)1/RConn1
